simulink model "MoHinh_NhanDang_Cau1"  (R2018a)
settings: Solver=FixedStepAuto  StartTime=0.0  StopTime=100.0  FixedStep=0.1  RelTol=1e-3
values from neighbouring files (symbols this model uses):
  b1 = 0.3    [thongso_cau1.m]
  k1 = 0.8    [thongso_cau1.m]
  m1 = 1.5    [thongso_cau1.m]
settings Model: OrderedModelArguments=off  Creator=20151  LastModifiedBy=20151
settings DataIOCC: ReturnWorkspaceOutputs=on
settings DebuggingCC: UnconnectedInputMsg=none  UnconnectedOutputMsg=none  UnconnectedLineMsg=none  SFMachineParentedDataDiag=error
settings SFSimCC: SimUseLocalCustomCode=on
settings RTWCC: RTWUseLocalCustomCode=on

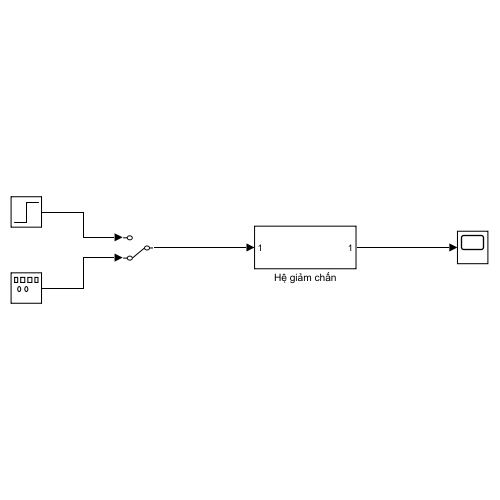
[thumbnail: Simulink's stored preview of the top-level diagram]
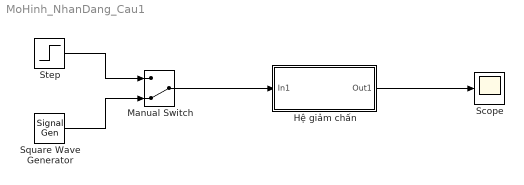
== system MoHinh_NhanDang_Cau1 ==
  Hệ giảm chấn : Subsystem
  Manual Switch : ManualSwitch  CurrentSetting=0
  Scope : Scope
  Square Wave Generator : SignalGenerator  WaveForm=random  Amplitude=20  Frequency=10  Units=rad/sec
  Step : Step  SampleTime=0.1
  wires:
  Step/1 -> Manual Switch/1
  Square Wave Generator/1 -> Manual Switch/2
  Hệ giảm chấn/1(Out1) -> Scope/1
  Manual Switch/1 -> Hệ giảm chấn/1(In1)

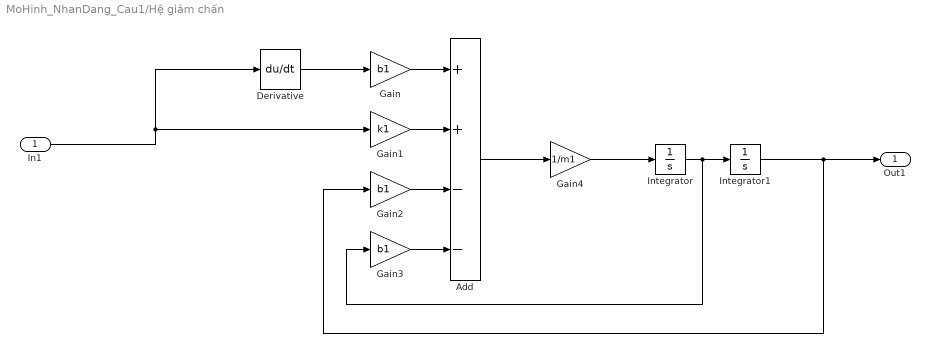
== system MoHinh_NhanDang_Cau1/Hệ giảm chấn ==
  In1 : Inport
  Add : Sum  Inputs=++--
  Derivative : Derivative
  Gain : Gain  Gain=b1
  Gain1 : Gain  Gain=k1
  Gain2 : Gain  Gain=b1
  Gain3 : Gain  Gain=b1
  Gain4 : Gain  Gain=1/m1
  Integrator : Integrator
  Integrator1 : Integrator
  Out1 : Outport
  wires:
  Gain/1 -> Add/1
  Gain1/1 -> Add/2
  Gain2/1 -> Add/3
  Gain3/1 -> Add/4
  Add/1 -> Gain4/1
  Derivative/1 -> Gain/1
  Gain4/1 -> Integrator/1
  Integrator/1 -> Gain3/1, Integrator1/1
  Integrator1/1 -> Gain2/1, Out1/1
  In1/1 -> Gain1/1, Derivative/1
